simulink model "State_space (1)"  (R2013a)
settings: Solver=ode45  StartTime=0.0  StopTime=10.0  RelTol=1e-3
values from neighbouring files (symbols this model uses):
  K = sigma * A*P*inv(s)    [Brid_code.m]    (also in Kalman_Filter.m = A_d*P*inv(s))
undefined symbols (not defined in the file or in its folder): A_d, B_d, C_d, D_d
libraries: simulink x1
settings Model: Creator=user  LastModifiedBy=user

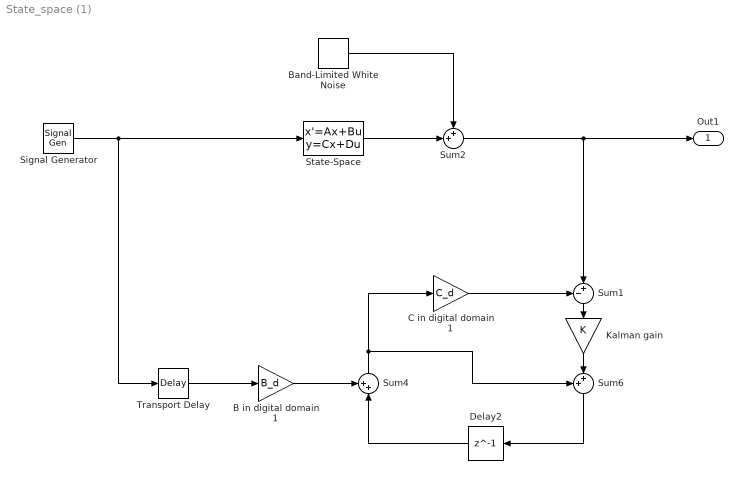
== system State_space (1) ==
  B in digital domain 1 : Gain  Gain=B_d
  Band-Limited White Noise : simulink/Sources/Band-Limited White Noise  Cov=[0.1]  Ts=0.1  seed=[23341]
  C in digital domain 1 : Gain  Gain=C_d
  Delay2 : Delay  DelayLength=1  InitialCondition=0
  Kalman gain : Gain  Gain=K
  Signal Generator : SignalGenerator
  State-Space : StateSpace  A=A_d  B=B_d  C=C_d  D=D_d
  Sum1 : Sum  Inputs=-+|
  Sum2 : Sum  Inputs=++|
  Sum4 : Sum  Inputs=++|
  Sum6 : Sum  Inputs=++|
  Transport Delay : TransportDelay
  Out1 : Outport
  wires:
  Signal Generator/1 -> Transport Delay/1, State-Space/1
  State-Space/1 -> Sum2/2
  Band-Limited White Noise/1 -> Sum2/1
  C in digital domain 1/1 -> Sum1/1
  Sum1/1 -> Kalman gain/1
  Sum4/1 -> Sum6/1, C in digital domain 1/1
  Kalman gain/1 -> Sum6/2
  Delay2/1 -> Sum4/2
  Sum6/1 -> Delay2/1
  Sum2/1 -> Sum1/2, Out1/1
  Transport Delay/1 -> B in digital domain 1/1
  B in digital domain 1/1 -> Sum4/1
